simulink model "ozoncc_m"  (Simulink 8.5)
settings: Solver=ode45  StartTime=0.0  StopTime=10.0  RelTol=1e-3
values from neighbouring files (symbols this model uses):
  U = st_Varia('LongNames')    [ozoncc_i.m]
  x0 = [O3*ones(NumCel,1);zeros(NumCel,1);UV254*ones(NumCel,1);zeros(NumCel,1);EC*ones(NumCel,1);zeros(NumCel,1)]    [ozoncc_i.m]    (also in ozoncc_s.m = x0)
undefined symbols (not defined in the file or in its folder): B
settings Model: Creator=M.Sparnaaij  LastModifiedBy=Martijn
settings DataIOCC: SignalLoggingName=sigsOut
settings DebuggingCC: SaveWithParameterizedLinksMsg=none  SignalResolutionControl=TryResolveAllWithWarning  MultiTaskDSMMsg=warning  MultiTaskCondExecSysMsg=none  FcnCallInpInsideContextMsg=EnableAllAsWarning  StrictBusMsg=None
settings HardwareCC: TargetUnknown=on

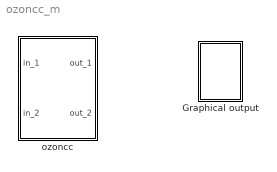
== system ozoncc_m ==
  Graphical output : Subsystem
      settings: OpenFcn=ozoncc_g
      mask Display:
      | plot(0,0,100,100,[80,20,20],[20,20,80],[80,69,60,52,45,39,33,28,24,20],[65,65,64,61,57,52,45,37,30,20])
      | disp('');
      | text(100,100,'ozoncc', 'horizontalAlignment', 'right', 'verticalAlignment', 'top');
  ozoncc : Subsystem
      mask init:
      | filenaam='.\StimelaData\ozon_reactor_BC.mat';
      | 
      | [Pn,Fn,Fext]=Fileprop(filenaam);
      | 
      | errstr = st_UniqName(filenaam,'filenaam=''','SubSystem','OpenFcn');
      | if errstr, error([errstr 'The filename "' filenaam '" is already in use. Choose a different filename.']), end
      | 
      | P = ozoncc_p(filenaam);
      | [B,x0,U]=ozoncc_i(filenaam);
      settings: OpenFcn=|
      | filenaam='.\StimelaData\ozon_reactor_BC.mat';
      | st_ParameterInput('init',gcb,filenaam,'ozoncc');
      mask Display:
      | plot(0,0,100,100,[80,80,20,20],[80,20,20,80],[30,70,70,30,30],[31,31,29,29,31],[35,35],[38,35],[35,35],[48,45],[35,35],[58,55],[35,35],[68,65],[40,40],[41,38],[40,40],[51,48],[40,40],[61,58],[40,40],[71,68],[45,45],[34,31],[45,45],[44,41],[45,45],[54,51],[45,45],[64,61],[45,45],[74,71],[50,50],[38,35],[50,50],[48,45],[50,50],[58,55],[50,50],[68,65],[55,55],[41,38],[55,55],[51,48],[55,55],[61,58],[55,55],[71,68],[60,60],[34,31],[60,60],[44,41],[60,60],[54,51],[60,60],[64,61],[60,60],[74,71],[65,65],[38,35],[65,65],[48,45],[65,65],[58,55],[65,65],[68,65])
      | disp('')
      | text(50,50,'ozoncc', 'horizontalAlignment', 'center', 'verticalAlignment', 'middle');
      | text(50,0,Fn, 'horizontalAlignment', 'center', 'verticalAlignment', 'base');

== system ozoncc_m/Graphical output ==
  note: plotten

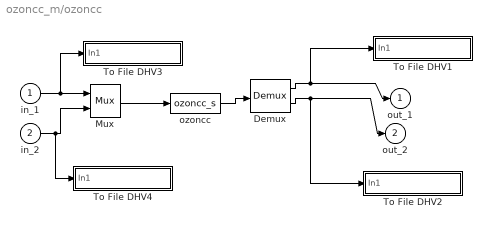
== system ozoncc_m/ozoncc ==
  in_1 : Inport
  in_2 : Inport  Port=2
  Demux : Demux  Outputs=[U.Number B.Measurements]
  Mux : Mux  Inputs=[U.Number B.Setpoints]
  To File DHV1 : Subsystem  mask(To File DHV){naam=[filenaam(1:length(filenaam)-4) '_out.sti']}
      mask prompts: naam "Naam van bestand"
      mask init:
      | set_param([gcb '/To File'],'Filename',naam);
      mask Display: disp(naam)
  To File DHV2 : Subsystem  mask(To File DHV){naam=[filenaam(1:length(filenaam)-4) '_EM.sti']}
      mask prompts: naam "Naam van bestand"
      mask init:
      | set_param([gcb '/To File'],'Filename',naam);
      mask Display: disp(naam)
  To File DHV3 : Subsystem  mask(To File DHV){naam=[filenaam(1:length(filenaam)-4) '_in.sti']}
      mask prompts: naam "Naam van bestand"
      mask init:
      | set_param([gcb '/To File'],'Filename',naam);
      mask Display: disp(naam)
  To File DHV4 : Subsystem  mask(To File DHV){naam=[filenaam(1:length(filenaam)-4) '_ES.sti']}
      mask prompts: naam "Naam van bestand"
      mask init:
      | set_param([gcb '/To File'],'Filename',naam);
      mask Display: disp(naam)
  ozoncc : S-Function  FunctionName=ozoncc_s  Parameters=B,x0,U,P
  out_1 : Outport  InitialOutput=0
  out_2 : Outport  Port=2  InitialOutput=0
  wires:
  in_2/1 -> To File DHV4/1(In1), Mux/2
  Mux/1 -> ozoncc/1
  in_1/1 -> To File DHV3/1(In1), Mux/1
  ozoncc/1 -> Demux/1
  Demux/1 -> To File DHV1/1(In1), out_1/1
  Demux/2 -> To File DHV2/1(In1), out_2/1

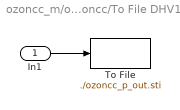
== system ozoncc_m/ozoncc/To File DHV1 ==
  In1 : Inport
  To File : ToFile  Filename=./ozoncc_p_out.sti  MatrixName=ozonccout
  wires:
  In1/1 -> To File/1

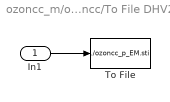
== system ozoncc_m/ozoncc/To File DHV2 ==
  In1 : Inport
  To File : ToFile  Filename=./ozoncc_p_EM.sti  MatrixName=ozonccEM
  wires:
  In1/1 -> To File/1

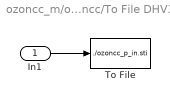
== system ozoncc_m/ozoncc/To File DHV3 ==
  In1 : Inport
  To File : ToFile  Filename=./ozoncc_p_in.sti  MatrixName=ozonccin
  wires:
  In1/1 -> To File/1

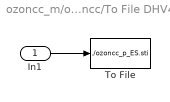
== system ozoncc_m/ozoncc/To File DHV4 ==
  In1 : Inport
  To File : ToFile  Filename=./ozoncc_p_ES.sti  MatrixName=ozonccES
  wires:
  In1/1 -> To File/1
